simulink model "pend_sim"  (R2024a)
settings: Solver=FixedStepAuto  StartTime=0.0  StopTime=10  FixedStep=0.01  RelTol=1e-3
InitFcn:
  | pend_parameters;
values from neighbouring files (symbols this model uses):
  A = [0 1 ; -g/l  -r/(m*l^2)]    [pend_parameters.m]
  B = [0 ; 1/(m*l^2)]    [pend_parameters.m]
  C = [1 0 ; 0 1]    [pend_parameters.m]
  D = 0    [pend_parameters.m]
  g = 9.81    [pend_parameters.m]
  l = 0.2    [pend_parameters.m]
  m = 1    [pend_parameters.m]
  r = 0.02    [pend_parameters.m]
  theta_0 = 1.3    [pend_parameters.m]
  thetadot_0 = 0    [pend_parameters.m]
settings Model: Creator=vcichella  LastModifiedBy=vcichella

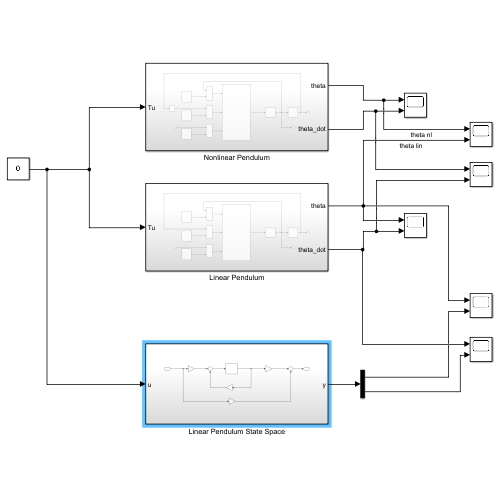
[thumbnail: Simulink's stored preview of the top-level diagram]
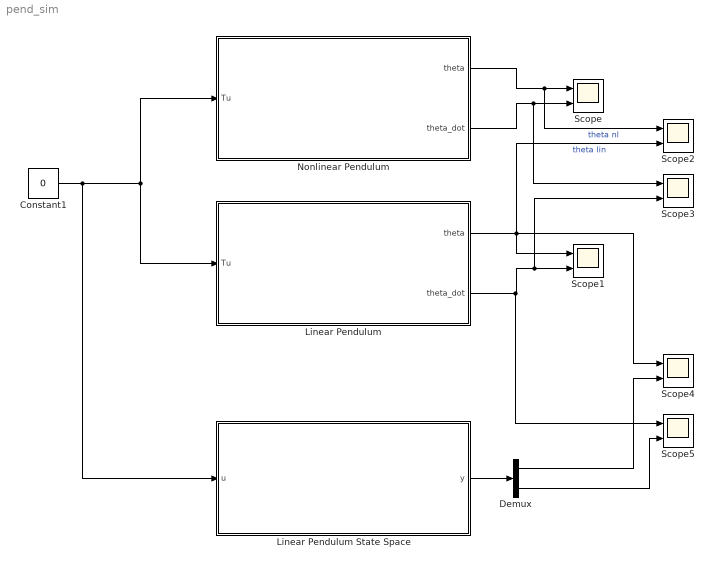
== system pend_sim ==
  Constant1 : Constant  Value=0
  Demux : Demux  Outputs=2
  Linear Pendulum : Subsystem
  Linear Pendulum State Space : Subsystem
  Nonlinear Pendulum : Subsystem
  Scope{,1..5} (6 alike) : Scope  NumInputPorts=2
  wires:
  Nonlinear Pendulum/1(theta) -> Scope2/1, Scope/1  "theta nl"
  Nonlinear Pendulum/2(theta_dot) -> Scope3/1, Scope/2
  Linear Pendulum/2(theta_dot) -> Scope5/1, Scope3/2, Scope1/2
  Linear Pendulum/1(theta) -> Scope4/1, Scope2/2, Scope1/1  "theta lin"
  Constant1/1 -> Linear Pendulum State Space/1(u), Nonlinear Pendulum/1(Tu), Linear Pendulum/1(Tu)
  Linear Pendulum State Space/1(y) -> Demux/1
  Demux/1 -> Scope4/2
  Demux/2 -> Scope5/2

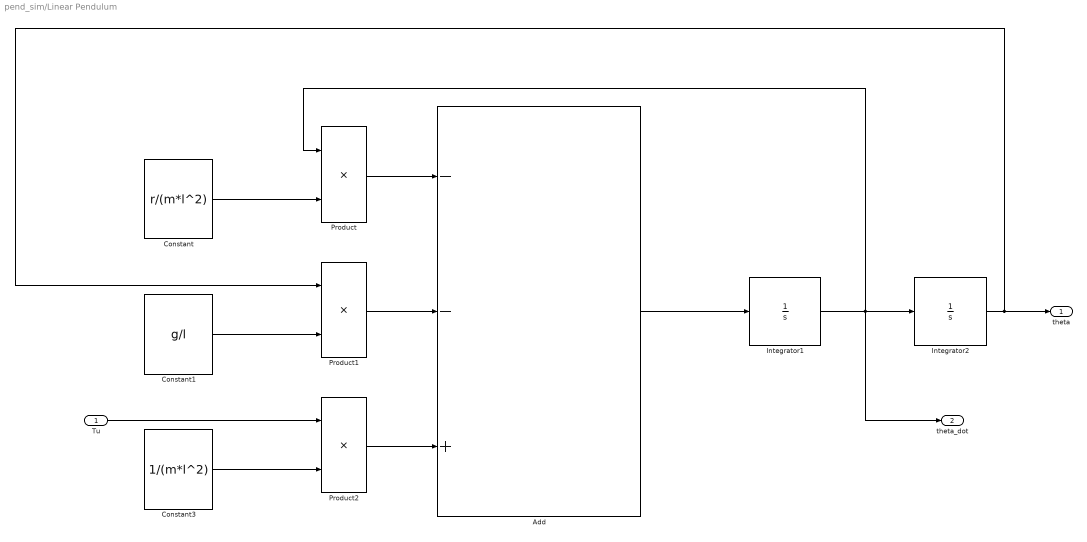
== system pend_sim/Linear Pendulum ==
  Tu : Inport
  Add : Sum  Inputs=--+
  Constant : Constant  Value=r/(m*l^2)
  Constant1 : Constant  Value=g/l
  Constant3 : Constant  Value=1/(m*l^2)
  Integrator1 : Integrator  InitialCondition=thetadot_0
  Integrator2 : Integrator  InitialCondition=theta_0
  Product : Product
  Product1 : Product
  Product2 : Product
  theta : Outport
  theta_dot : Outport  Port=2
  wires:
  Constant3/1 -> Product2/2
  Product2/1 -> Add/3
  Tu/1 -> Product2/1
  Add/1 -> Integrator1/1
  Product1/1 -> Add/2
  Product/1 -> Add/1
  Constant/1 -> Product/2
  Integrator2/1 -> Product1/1, theta/1
  Integrator1/1 -> Integrator2/1, Product/1, theta_dot/1
  Constant1/1 -> Product1/2

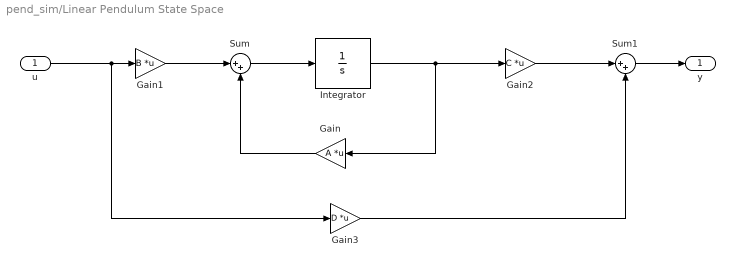
== system pend_sim/Linear Pendulum State Space ==
  u : Inport
  Gain : Gain  Gain=A  Multiplication=Matrix(K*u)
  Gain1 : Gain  Gain=B  Multiplication=Matrix(K*u)
  Gain2 : Gain  Gain=C  Multiplication=Matrix(K*u)
  Gain3 : Gain  Gain=D  Multiplication=Matrix(K*u)
  Integrator : Integrator  InitialCondition=[theta_0; thetadot_0]
  Sum : Sum  Inputs=|++
  Sum1 : Sum  Inputs=|++
  y : Outport
  wires:
  Gain/1 -> Sum/2
  Gain1/1 -> Sum/1
  Sum/1 -> Integrator/1
  Sum1/1 -> y/1
  Gain2/1 -> Sum1/1
  Integrator/1 -> Gain2/1, Gain/1
  u/1 -> Gain3/1, Gain1/1
  Gain3/1 -> Sum1/2

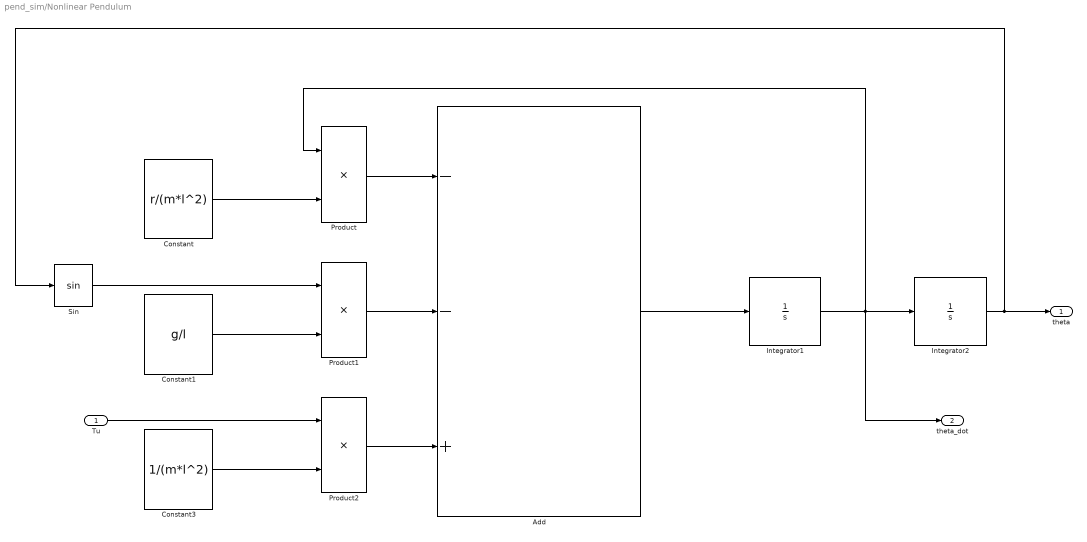
== system pend_sim/Nonlinear Pendulum ==
  Tu : Inport
  Add : Sum  Inputs=--+
  Constant : Constant  Value=r/(m*l^2)
  Constant1 : Constant  Value=g/l
  Constant3 : Constant  Value=1/(m*l^2)
  Integrator1 : Integrator  InitialCondition=thetadot_0
  Integrator2 : Integrator  InitialCondition=theta_0
  Product : Product
  Product1 : Product
  Product2 : Product
  Sin : Trigonometry
  theta : Outport
  theta_dot : Outport  Port=2
  wires:
  Constant1/1 -> Product1/2
  Integrator1/1 -> theta_dot/1, Product/1, Integrator2/1
  Sin/1 -> Product1/1
  Constant/1 -> Product/2
  Product/1 -> Add/1
  Product1/1 -> Add/2
  Add/1 -> Integrator1/1
  Integrator2/1 -> theta/1, Sin/1
  Tu/1 -> Product2/1
  Product2/1 -> Add/3
  Constant3/1 -> Product2/2
